simulink model "circuit_Rasp_full_2_only_res"  (R2018b)
settings: Solver=VariableStepAuto  StartTime=0.0  StopTime=10.0  RelTol=1e-3
libraries: nesl_utility x27, fl_lib x23, pe_lib x20
settings Model: Creator=giovannirenda  LastModifiedBy=giovannirenda
settings DebuggingCC: LibraryContextMissingDiagnostic=none
settings SFSimCC: SimUseLocalCustomCode=off
settings RTWCC: RTWUseLocalCustomCode=off

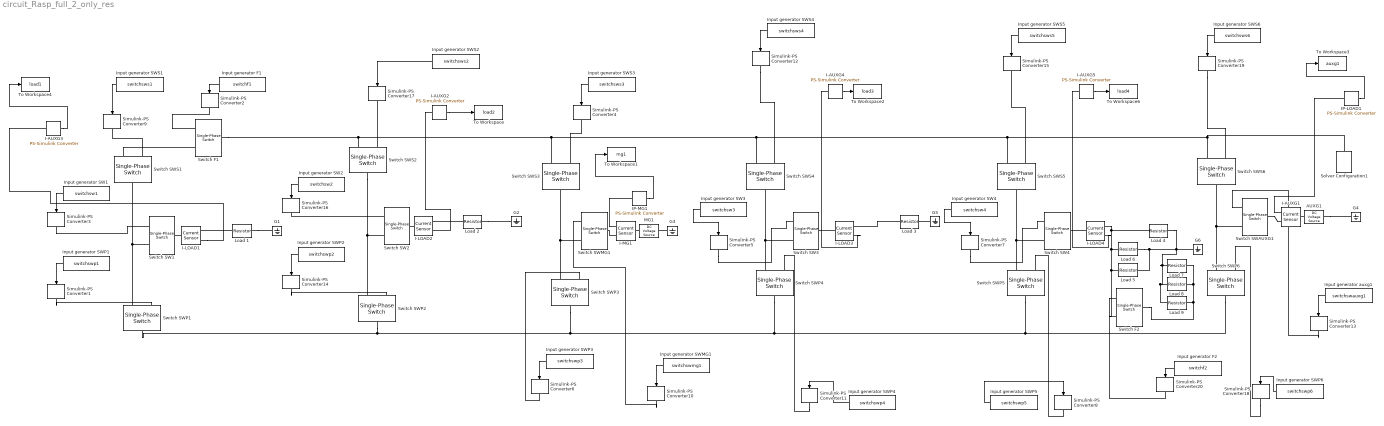
== system circuit_Rasp_full_2_only_res ==
  AUXG1 : fl_lib/Electrical/Electrical Sources/DC Voltage Source  v0=3.3 V
  G{1..6} (6 alike) : fl_lib/Electrical/Electrical Elements/Electrical Reference
  I-AUXG1 : fl_lib/Electrical/Electrical Sensors/Current Sensor
  I-AUXG{2..5} (4 alike) : nesl_utility/PS-Simulink Converter  PhysicalDomain=network_engine_domain  SubClassName=ps_output  LeftPortType=input  RightPortType=output  PseudoPeriodic=off  Frequencies=[]  Unit=A  AffineConversion=off
  I-LOAD{1..4} (4 alike) : fl_lib/Electrical/Electrical Sensors/Current Sensor
  I-MG1 : fl_lib/Electrical/Electrical Sensors/Current Sensor
  IP-LOAD1 : nesl_utility/PS-Simulink Converter  PhysicalDomain=network_engine_domain  SubClassName=ps_output  LeftPortType=input  RightPortType=output  PseudoPeriodic=off  Frequencies=[]  Unit=A  AffineConversion=off
  IP-MG1 : nesl_utility/PS-Simulink Converter  PhysicalDomain=network_engine_domain  SubClassName=ps_output  LeftPortType=input  RightPortType=output  PseudoPeriodic=off  Frequencies=[]  Unit=A  AffineConversion=off
  Input generator F1 : FromWorkspace  VariableName=switchf1  SampleTime=1
  Input generator F2 : FromWorkspace  VariableName=switchf2  SampleTime=1
  Input generator SW1 : FromWorkspace  VariableName=switchsw1  SampleTime=1
  Input generator SW2 : FromWorkspace  VariableName=switchsw2  SampleTime=1
  Input generator SW3 : FromWorkspace  VariableName=switchsw3  SampleTime=1
  Input generator SW4 : FromWorkspace  VariableName=switchsw4  SampleTime=1
  Input generator SWMG1 : FromWorkspace  VariableName=switchswmg1  SampleTime=1
  Input generator SWP1 : FromWorkspace  VariableName=switchswp1  SampleTime=1
  Input generator SWP2 : FromWorkspace  VariableName=switchswp2  SampleTime=1
  Input generator SWP3 : FromWorkspace  VariableName=switchswp3  SampleTime=1
  Input generator SWP4 : FromWorkspace  VariableName=switchswp4  SampleTime=1
  Input generator SWP5 : FromWorkspace  VariableName=switchswp5  SampleTime=1
  Input generator SWP6 : FromWorkspace  VariableName=switchswp6  SampleTime=1
  Input generator SWS1 : FromWorkspace  VariableName=switchsws1  SampleTime=1
  Input generator SWS2 : FromWorkspace  VariableName=switchsws2  SampleTime=1
  Input generator SWS3 : FromWorkspace  VariableName=switchsws3  SampleTime=1
  Input generator SWS4 : FromWorkspace  VariableName=switchsws4  SampleTime=1
  Input generator SWS5 : FromWorkspace  VariableName=switchsws5  SampleTime=1
  Input generator SWS6 : FromWorkspace  VariableName=switchsws6  SampleTime=1
  Input generator auxg1 : FromWorkspace  VariableName=switchswauxg1  SampleTime=1
  Load 1 : fl_lib/Electrical/Electrical Elements/Resistor  R=12.7 Ohm  i_specify=off  i_priority=None  i=0 A  i_nominal_specify=off  i_nominal_unit=A  i_nominal_value=1  v_specify=off  v_priority=None  v=0 V  v_nominal_specify=off  v_nominal_unit=V  v_nominal_value=1
  Load 2 : fl_lib/Electrical/Electrical Elements/Resistor  R=12.7 Ohm  i_specify=off  i_priority=None  i=0 A  i_nominal_specify=off  i_nominal_unit=A  i_nominal_value=1  v_specify=off  v_priority=None  v=0 V  v_nominal_specify=off  v_nominal_unit=V  v_nominal_value=1
  Load 3 : fl_lib/Electrical/Electrical Elements/Resistor  R=91.67 Ohm  i_specify=off  i_priority=None  i=0 A  i_nominal_specify=off  i_nominal_unit=A  i_nominal_value=1  v_specify=off  v_priority=None  v=0 V  v_nominal_specify=off  v_nominal_unit=V  v_nominal_value=1
  Load 4 : fl_lib/Electrical/Electrical Elements/Resistor  R=550 Ohm  i_specify=off  i_priority=None  i=0 A  i_nominal_specify=off  i_nominal_unit=A  i_nominal_value=1  v_specify=off  v_priority=None  v=0 V  v_nominal_specify=off  v_nominal_unit=V  v_nominal_value=1
  Load {5..9} (5 alike) : fl_lib/Electrical/Electrical Elements/Resistor  R=220 Ohm  i_specify=off  i_priority=None  i=0 A  i_nominal_specify=off  i_nominal_unit=A  i_nominal_value=1  v_specify=off  v_priority=None  v=0 V  v_nominal_specify=off  v_nominal_unit=V  v_nominal_value=1
  MG1 : fl_lib/Electrical/Electrical Sources/DC Voltage Source  v0=3.3 V
  Simulink-PS Converter{1..20} (20 alike) : nesl_utility/Simulink-PS Converter  PhysicalDomain=network_engine_domain  SubClassName=ps_input  LeftPortType=input  RightPortType=output  PseudoPeriodic=off  Frequencies=[]  NoiseDistribution=none  NoiseParameters=[]  Unit=1  AffineConversion=off  FilteringAndDerivatives=zero  SimscapeFilterOrder=1  InputFilterTimeConstant=0.001  UdotUserProvided=1
  Solver Configuration1 : nesl_utility/Solver Configuration  PhysicalDomain=network_engine_domain  SubClassName=solver  LeftPortType=input  RightPortType=generic  Tones=[]  Harmonics=[]  SimulateNoise=off  Profile=off  UseLocalSampling=off  EnableSwitchedLinearOptims=on  FrequencyDomain=off  UseCCode=off  RelTol=0.001  AbsTol=1e-06  MinStep=1e-09  ToWorkspace=off  RevertToSquareIcSolve=off  NumHomotopyIterations=100  PhasorMode=off  PhasorModeNumHarmonics=1  DoDC=off  ResidualTolerance=1e-09  UseLocalSolver=off  LocalSolverChoice=NE_BACKWARD_EULER_ADVANCER  LocalSolverSampleTime=0.001  DoFixedCost=off  MaxNonlinIter=3  MaxModeIter=2  LinearAlgebra=Sparse  EquationFormulation=NE_TIME_EF  DelaysMemoryBudget=1024  AutomaticFiltering=on  FilteringTimeConstant=0.001  PartitionStorageMethod=AS_NEEDED  PartitionMemoryBudget=1024
  Switch F1 : pe_lib/Switches & Breakers/Fundamental Components/Single-Phase Switch  R_closed=0.001 Ohm  G_open=1e-6 1/Ohm  threshold=0 V
      settings: SourceProductName=Simscape Electrical  SourceProductBaseCode=PS
  Switch F2 : pe_lib/Switches & Breakers/Fundamental Components/Single-Phase Switch  R_closed=0.001 Ohm  G_open=1e-6 1/Ohm  threshold=0 V
      settings: SourceProductName=Simscape Electrical  SourceProductBaseCode=PS
  Switch SW{1..4} (4 alike) : pe_lib/Switches & Breakers/Fundamental Components/Single-Phase Switch  R_closed=0.001 Ohm  G_open=1e-6 1/Ohm  threshold=0 V
      settings: SourceProductName=Simscape Electrical  SourceProductBaseCode=PS
  Switch SWAUXG1 : pe_lib/Switches & Breakers/Fundamental Components/Single-Phase Switch  R_closed=0.001 Ohm  G_open=1e-6 1/Ohm  threshold=0 V
      settings: SourceProductName=Simscape Electrical  SourceProductBaseCode=PS
  Switch SWMG1 : pe_lib/Switches & Breakers/Fundamental Components/Single-Phase Switch  R_closed=0.001 Ohm  G_open=1e-6 1/Ohm  threshold=0 V
      settings: SourceProductName=Simscape Electrical  SourceProductBaseCode=PS
  Switch SWP{1..6} (6 alike) : pe_lib/Switches & Breakers/Fundamental Components/Single-Phase Switch  R_closed=0.001 Ohm  G_open=1e-6 1/Ohm  threshold=0 V
      settings: SourceProductName=Simscape Electrical  SourceProductBaseCode=PS
  Switch SWS{1..6} (6 alike) : pe_lib/Switches & Breakers/Fundamental Components/Single-Phase Switch  R_closed=0.001 Ohm  G_open=1e-6 1/Ohm  threshold=0 V
      settings: SourceProductName=Simscape Electrical  SourceProductBaseCode=PS
  To Workspace : ToWorkspace  VariableName=load2  SampleTime=1
      settings: Save2DSignal=2-D array (concatenate along first dimension)
  To Workspace1 : ToWorkspace  VariableName=mg1  SampleTime=1
      settings: Save2DSignal=2-D array (concatenate along first dimension)
  To Workspace2 : ToWorkspace  VariableName=load3  SampleTime=1
      settings: Save2DSignal=2-D array (concatenate along first dimension)
  To Workspace3 : ToWorkspace  VariableName=auxg1  SampleTime=1
      settings: Save2DSignal=2-D array (concatenate along first dimension)
  To Workspace4 : ToWorkspace  VariableName=load1  SampleTime=1
      settings: Save2DSignal=2-D array (concatenate along first dimension)
  To Workspace6 : ToWorkspace  VariableName=load4  SampleTime=1
  wires:
  Input generator SWS1/1 -> Simulink-PS Converter9/1
  Input generator SWP1/1 -> Simulink-PS Converter1/1
  Input generator F1/1 -> Simulink-PS Converter2/1
  Input generator SW1/1 -> Simulink-PS Converter3/1
  Input generator SWS3/1 -> Simulink-PS Converter4/1
  Input generator SWP3/1 -> Simulink-PS Converter6/1
  Input generator SWMG1/1 -> Simulink-PS Converter10/1
  I-AUXG3/1 -> To Workspace4/1
  IP-MG1/1 -> To Workspace1/1
  IP-LOAD1/1 -> To Workspace3/1
  Input generator auxg1/1 -> Simulink-PS Converter13/1
  Input generator SWP2/1 -> Simulink-PS Converter14/1
  Input generator SW2/1 -> Simulink-PS Converter16/1
  Input generator SWS2/1 -> Simulink-PS Converter17/1
  I-AUXG2/1 -> To Workspace/1
  I-AUXG4/1 -> To Workspace2/1
  Input generator SWS4/1 -> Simulink-PS Converter12/1
  Input generator SWP4/1 -> Simulink-PS Converter11/1
  Input generator SW3/1 -> Simulink-PS Converter5/1
  Input generator SW4/1 -> Simulink-PS Converter7/1
  Input generator SWP5/1 -> Simulink-PS Converter8/1
  Input generator SWS5/1 -> Simulink-PS Converter15/1
  I-AUXG5/1 -> To Workspace6/1
  Input generator SWP6/1 -> Simulink-PS Converter18/1
  Input generator SWS6/1 -> Simulink-PS Converter19/1
  Input generator F2/1 -> Simulink-PS Converter20/1
  connections:
  Switch SW1/LConn2 -- Switch SWP1/LConn2 -- Switch SWS1/RConn1
  Load 1/RConn1 -- G1/LConn1
  G3/LConn1 -- MG1/RConn1
  Switch SWS6/LConn2 -- Solver Configuration1/RConn1 -- Switch SWS4/LConn2 -- Switch SWS3/LConn2 -- Switch SWS2/LConn2 -- Switch F1/RConn1 -- Switch SWS5/LConn2
  Switch SWP1/RConn1 -- Switch SWP2/RConn1 -- Switch SWP6/RConn1 -- Switch SWP5/RConn1 -- Switch SWP4/RConn1 -- Switch SWP3/RConn1
  Switch SWS1/LConn2 -- Switch F1/LConn2
  Switch SWS1/LConn1 -- Simulink-PS Converter9/RConn1
  Simulink-PS Converter1/RConn1 -- Switch SWP1/LConn1
  Simulink-PS Converter2/RConn1 -- Switch F1/LConn1
  Simulink-PS Converter3/RConn1 -- Switch SW1/LConn1
  Switch SWS3/LConn1 -- Simulink-PS Converter4/RConn1
  Simulink-PS Converter6/RConn1 -- Switch SWP3/LConn1
  Simulink-PS Converter10/RConn1 -- Switch SWMG1/LConn1
  I-LOAD1/RConn1 -- I-AUXG3/LConn1
  I-MG1/RConn2 -- Switch SWMG1/RConn1
  I-MG1/LConn1 -- MG1/LConn1
  I-LOAD1/LConn1 -- Switch SW1/RConn1
  IP-MG1/LConn1 -- I-MG1/RConn1
  I-AUXG1/LConn1 -- AUXG1/LConn1
  AUXG1/RConn1 -- G4/LConn1
  Switch SWAUXG1/RConn1 -- I-AUXG1/RConn2
  IP-LOAD1/LConn1 -- I-AUXG1/RConn1
  Simulink-PS Converter13/RConn1 -- Switch SWAUXG1/LConn1
  Load 1/LConn1 -- I-LOAD1/RConn2
  Switch SWS2/RConn1 -- Switch SW2/LConn2 -- Switch SWP2/LConn2
  Load 2/RConn1 -- G2/LConn1
  Load 2/LConn1 -- I-LOAD2/RConn2
  Switch SW2/LConn1 -- Simulink-PS Converter16/RConn1
  Switch SWS2/LConn1 -- Simulink-PS Converter17/RConn1
  I-LOAD2/LConn1 -- Switch SW2/RConn1
  I-AUXG2/LConn1 -- I-LOAD2/RConn1
  Simulink-PS Converter14/RConn1 -- Switch SWP2/LConn1
  Switch SWMG1/LConn2 -- Switch SWS3/RConn1 -- Switch SWP3/LConn2
  Switch SWP4/LConn2 -- Switch SWS4/RConn1 -- Switch SW3/LConn2
  G5/LConn1 -- Load 3/RConn1
  I-LOAD3/LConn1 -- Switch SW3/RConn1
  Load 3/LConn1 -- I-LOAD3/RConn2
  I-LOAD3/RConn1 -- I-AUXG4/LConn1
  Simulink-PS Converter12/RConn1 -- Switch SWS4/LConn1
  Simulink-PS Converter11/RConn1 -- Switch SWP4/LConn1
  Simulink-PS Converter5/RConn1 -- Switch SW3/LConn1
  Switch SWP5/LConn2 -- Switch SWS5/RConn1 -- Switch SW4/LConn2
  Load 9/LConn1 -- Load 4/RConn1 -- G6/LConn1 -- Load 6/RConn1 -- Load 5/RConn1 -- Load 7/LConn1 -- Load 8/LConn1
  Switch F2/LConn2 -- Load 5/LConn1 -- Load 6/LConn1 -- Load 4/LConn1 -- I-LOAD4/RConn2
  Simulink-PS Converter7/RConn1 -- Switch SW4/LConn1
  I-LOAD4/LConn1 -- Switch SW4/RConn1
  Simulink-PS Converter8/RConn1 -- Switch SWP5/LConn1
  Switch SWS5/LConn1 -- Simulink-PS Converter15/RConn1
  I-LOAD4/RConn1 -- I-AUXG5/LConn1
  Switch SWAUXG1/LConn2 -- Switch SWS6/RConn1 -- Switch SWP6/LConn2
  Simulink-PS Converter18/RConn1 -- Switch SWP6/LConn1
  Simulink-PS Converter19/RConn1 -- Switch SWS6/LConn1
  Load 7/RConn1 -- Switch F2/RConn1 -- Load 9/RConn1 -- Load 8/RConn1
  Simulink-PS Converter20/RConn1 -- Switch F2/LConn1
